simulink model "WorkingModel"  (R2023b)
settings: Solver=FixedStepDiscrete  StartTime=0.0  StopTime=param_sim_time  FixedStep=1/fs  MaxStep=1/fs  RelTol=1e-3
undefined symbols (not defined in the file): analyses, fdesignblkfcn, fs, gcbh, param_tot_samples
libraries: dspstat3 x13, SCGAnalysis_SignalGenerationLib x2
(part 10 of 20)

== system WorkingModel/SCG Analysis/Enabled SCG Analysis Subsystem/All Signals Signal Metric Characterization/SCG S2 3DMechAxis Signal Metric Characterization/Average Signal-to-Noise Ratio Calculator/Average S2 Signal-to-Noise Ratio ==
  r_pos : Inport
  scg_signal : Inport  Port=2
  " " : Constant  Value=s2snr_flag
  Average S2 SNR Calculator : MATLAB Function  TreatAsAtomicUnit=on
  Constant : Constant  Value=fs
  Constant1 : Constant  Value=0
  Switch : Switch  Criteria=u2 > Threshold  AllowDiffInputSizes=on  SaturateOnIntegerOverflow=off  InputSameDT=off
  average_s2snr : Outport
  wires:
  r_pos/1 -> Switch/1
  Constant1/1 -> Switch/3
  " "/1 -> Switch/2
  Constant/1 -> Average S2 SNR Calculator/1(fs)
  scg_signal/1 -> Average S2 SNR Calculator/3(scg_signal)
  Switch/1 -> Average S2 SNR Calculator/2(r_pos)
  Average S2 SNR Calculator/1(average_s2_snr) -> average_s2snr/1

== system WorkingModel/SCG Analysis/Enabled SCG Analysis Subsystem/All Signals Signal Metric Characterization/SCG S2 3DMechAxis Signal Metric Characterization/Average Signal-to-Noise Ratio Calculator/Average S2X Signal-to-Noise Ratio ==
  r_pos : Inport
  scg_signal : Inport  Port=2
  " " : Constant  Value=s2xsnr_flag
  Average S2X SNR Calculator : MATLAB Function  TreatAsAtomicUnit=on
  Constant : Constant  Value=fs
  Constant1 : Constant  Value=0
  Switch : Switch  Criteria=u2 > Threshold  AllowDiffInputSizes=on  SaturateOnIntegerOverflow=off  InputSameDT=off
  average_s2Xsnr : Outport
  wires:
  r_pos/1 -> Switch/1
  Constant1/1 -> Switch/3
  " "/1 -> Switch/2
  Constant/1 -> Average S2X SNR Calculator/1(fs)
  scg_signal/1 -> Average S2X SNR Calculator/3(scg_signal)
  Switch/1 -> Average S2X SNR Calculator/2(r_pos)
  Average S2X SNR Calculator/1(average_s2x_snr) -> average_s2Xsnr/1

== system WorkingModel/SCG Analysis/Enabled SCG Analysis Subsystem/All Signals Signal Metric Characterization/SCG Systolic 3DAntiMechAxis Signal Metric Characterization/Average Signal-to-Noise Ratio Calculator/Average S1 Signal-to-Noise Ratio ==
  r_pos : Inport
  scg_signal : Inport  Port=2
  " " : Constant  Value=s1snr_flag
  Average S1 SNR Calculator : MATLAB Function  TreatAsAtomicUnit=on
  Constant : Constant  Value=fs
  Constant1 : Constant  Value=0
  Switch : Switch  Criteria=u2 > Threshold  AllowDiffInputSizes=on  SaturateOnIntegerOverflow=off  InputSameDT=off
  average_s1snr : Outport
  wires:
  scg_signal/1 -> Average S1 SNR Calculator/3(scg_signal)
  Average S1 SNR Calculator/1(average_s1_snr) -> average_s1snr/1
  Constant/1 -> Average S1 SNR Calculator/1(fs)
  " "/1 -> Switch/2
  Switch/1 -> Average S1 SNR Calculator/2(r_pos)
  r_pos/1 -> Switch/1
  Constant1/1 -> Switch/3

== system WorkingModel/SCG Analysis/Enabled SCG Analysis Subsystem/All Signals Signal Metric Characterization/SCG Systolic 3DAntiMechAxis Signal Metric Characterization/Average Signal-to-Noise Ratio Calculator/Average S1X Signal-to-Noise Ratio ==
  r_pos : Inport
  scg_signal : Inport  Port=2
  " " : Constant  Value=s1xsnr_flag
  Average S1 SNR Amplitude Calculator : MATLAB Function  TreatAsAtomicUnit=on
  Constant : Constant  Value=fs
  Constant1 : Constant  Value=0
  Switch : Switch  Criteria=u2 > Threshold  AllowDiffInputSizes=on  SaturateOnIntegerOverflow=off  InputSameDT=off
  average_s1Xsnr : Outport
  wires:
  Average S1 SNR Amplitude Calculator/1(average_s1x_snr) -> average_s1Xsnr/1
  Switch/1 -> Average S1 SNR Amplitude Calculator/2(r_pos)
  scg_signal/1 -> Average S1 SNR Amplitude Calculator/3(scg_signal)
  Constant/1 -> Average S1 SNR Amplitude Calculator/1(fs)
  " "/1 -> Switch/2
  Constant1/1 -> Switch/3
  r_pos/1 -> Switch/1

== system WorkingModel/SCG Analysis/Enabled SCG Analysis Subsystem/All Signals Signal Metric Characterization/SCG Systolic 3DAntiMechAxis Signal Metric Characterization/Average Signal-to-Noise Ratio Calculator/Average S2 Signal-to-Noise Ratio ==
  r_pos : Inport
  scg_signal : Inport  Port=2
  " " : Constant  Value=s2snr_flag
  Average S2 SNR Calculator : MATLAB Function  TreatAsAtomicUnit=on
  Constant : Constant  Value=fs
  Constant1 : Constant  Value=0
  Switch : Switch  Criteria=u2 > Threshold  AllowDiffInputSizes=on  SaturateOnIntegerOverflow=off  InputSameDT=off
  average_s2snr : Outport
  wires:
  Average S2 SNR Calculator/1(average_s2_snr) -> average_s2snr/1
  Switch/1 -> Average S2 SNR Calculator/2(r_pos)
  scg_signal/1 -> Average S2 SNR Calculator/3(scg_signal)
  Constant/1 -> Average S2 SNR Calculator/1(fs)
  " "/1 -> Switch/2
  Constant1/1 -> Switch/3
  r_pos/1 -> Switch/1

== system WorkingModel/SCG Analysis/Enabled SCG Analysis Subsystem/All Signals Signal Metric Characterization/SCG Systolic 3DAntiMechAxis Signal Metric Characterization/Average Signal-to-Noise Ratio Calculator/Average S2X Signal-to-Noise Ratio ==
  r_pos : Inport
  scg_signal : Inport  Port=2
  " " : Constant  Value=s2xsnr_flag
  Average S2X SNR Calculator : MATLAB Function  TreatAsAtomicUnit=on
  Constant : Constant  Value=fs
  Constant1 : Constant  Value=0
  Switch : Switch  Criteria=u2 > Threshold  AllowDiffInputSizes=on  SaturateOnIntegerOverflow=off  InputSameDT=off
  average_s2Xsnr : Outport
  wires:
  Average S2X SNR Calculator/1(average_s2x_snr) -> average_s2Xsnr/1
  Switch/1 -> Average S2X SNR Calculator/2(r_pos)
  scg_signal/1 -> Average S2X SNR Calculator/3(scg_signal)
  Constant/1 -> Average S2X SNR Calculator/1(fs)
  " "/1 -> Switch/2
  Constant1/1 -> Switch/3
  r_pos/1 -> Switch/1

== system WorkingModel/SCG Analysis/Enabled SCG Analysis Subsystem/All Signals Signal Metric Characterization/SCG Systolic 3DMaxS1p2pProjection Signal Metric Characterization/Average Signal-to-Noise Ratio Calculator/Average S1 Signal-to-Noise Ratio ==
  r_pos : Inport
  scg_signal : Inport  Port=2
  " " : Constant  Value=s1snr_flag
  Average S1 SNR Calculator : MATLAB Function  TreatAsAtomicUnit=on
  Constant : Constant  Value=fs
  Constant1 : Constant  Value=0
  Switch : Switch  Criteria=u2 > Threshold  AllowDiffInputSizes=on  SaturateOnIntegerOverflow=off  InputSameDT=off
  average_s1snr : Outport
  wires:
  Constant1/1 -> Switch/3
  r_pos/1 -> Switch/1
  Switch/1 -> Average S1 SNR Calculator/2(r_pos)
  " "/1 -> Switch/2
  Constant/1 -> Average S1 SNR Calculator/1(fs)
  Average S1 SNR Calculator/1(average_s1_snr) -> average_s1snr/1
  scg_signal/1 -> Average S1 SNR Calculator/3(scg_signal)

== system WorkingModel/SCG Analysis/Enabled SCG Analysis Subsystem/All Signals Signal Metric Characterization/SCG Systolic 3DMaxS1p2pProjection Signal Metric Characterization/Average Signal-to-Noise Ratio Calculator/Average S1X Signal-to-Noise Ratio ==
  r_pos : Inport
  scg_signal : Inport  Port=2
  " " : Constant  Value=s1xsnr_flag
  Average S1 SNR Amplitude Calculator : MATLAB Function  TreatAsAtomicUnit=on
  Constant : Constant  Value=fs
  Constant1 : Constant  Value=0
  Switch : Switch  Criteria=u2 > Threshold  AllowDiffInputSizes=on  SaturateOnIntegerOverflow=off  InputSameDT=off
  average_s1Xsnr : Outport
  wires:
  r_pos/1 -> Switch/1
  Constant1/1 -> Switch/3
  " "/1 -> Switch/2
  Constant/1 -> Average S1 SNR Amplitude Calculator/1(fs)
  scg_signal/1 -> Average S1 SNR Amplitude Calculator/3(scg_signal)
  Switch/1 -> Average S1 SNR Amplitude Calculator/2(r_pos)
  Average S1 SNR Amplitude Calculator/1(average_s1x_snr) -> average_s1Xsnr/1

== system WorkingModel/SCG Analysis/Enabled SCG Analysis Subsystem/All Signals Signal Metric Characterization/SCG Systolic 3DMaxS1p2pProjection Signal Metric Characterization/Average Signal-to-Noise Ratio Calculator/Average S2 Signal-to-Noise Ratio ==
  r_pos : Inport
  scg_signal : Inport  Port=2
  " " : Constant  Value=s2snr_flag
  Average S2 SNR Calculator : MATLAB Function  TreatAsAtomicUnit=on
  Constant : Constant  Value=fs
  Constant1 : Constant  Value=0
  Switch : Switch  Criteria=u2 > Threshold  AllowDiffInputSizes=on  SaturateOnIntegerOverflow=off  InputSameDT=off
  average_s2snr : Outport
  wires:
  r_pos/1 -> Switch/1
  Constant1/1 -> Switch/3
  " "/1 -> Switch/2
  Constant/1 -> Average S2 SNR Calculator/1(fs)
  scg_signal/1 -> Average S2 SNR Calculator/3(scg_signal)
  Switch/1 -> Average S2 SNR Calculator/2(r_pos)
  Average S2 SNR Calculator/1(average_s2_snr) -> average_s2snr/1

== system WorkingModel/SCG Analysis/Enabled SCG Analysis Subsystem/All Signals Signal Metric Characterization/SCG Systolic 3DMaxS1p2pProjection Signal Metric Characterization/Average Signal-to-Noise Ratio Calculator/Average S2X Signal-to-Noise Ratio ==
  r_pos : Inport
  scg_signal : Inport  Port=2
  " " : Constant  Value=s2xsnr_flag
  Average S2X SNR Calculator : MATLAB Function  TreatAsAtomicUnit=on
  Constant : Constant  Value=fs
  Constant1 : Constant  Value=0
  Switch : Switch  Criteria=u2 > Threshold  AllowDiffInputSizes=on  SaturateOnIntegerOverflow=off  InputSameDT=off
  average_s2Xsnr : Outport
  wires:
  r_pos/1 -> Switch/1
  Constant1/1 -> Switch/3
  " "/1 -> Switch/2
  Constant/1 -> Average S2X SNR Calculator/1(fs)
  scg_signal/1 -> Average S2X SNR Calculator/3(scg_signal)
  Switch/1 -> Average S2X SNR Calculator/2(r_pos)
  Average S2X SNR Calculator/1(average_s2x_snr) -> average_s2Xsnr/1

== system WorkingModel/SCG Analysis/Enabled SCG Analysis Subsystem/All Signals Signal Metric Characterization/SCG Systolic 3DMechAxis Signal Metric Characterization/Average Signal-to-Noise Ratio Calculator/Average S1 Signal-to-Noise Ratio ==
  r_pos : Inport
  scg_signal : Inport  Port=2
  " " : Constant  Value=s1snr_flag
  Average S1 SNR Calculator : MATLAB Function  TreatAsAtomicUnit=on
  Constant : Constant  Value=fs
  Constant1 : Constant  Value=0
  Switch : Switch  Criteria=u2 > Threshold  AllowDiffInputSizes=on  SaturateOnIntegerOverflow=off  InputSameDT=off
  average_s1snr : Outport
  wires:
  Constant1/1 -> Switch/3
  r_pos/1 -> Switch/1
  Switch/1 -> Average S1 SNR Calculator/2(r_pos)
  " "/1 -> Switch/2
  Constant/1 -> Average S1 SNR Calculator/1(fs)
  Average S1 SNR Calculator/1(average_s1_snr) -> average_s1snr/1
  scg_signal/1 -> Average S1 SNR Calculator/3(scg_signal)

== system WorkingModel/SCG Analysis/Enabled SCG Analysis Subsystem/All Signals Signal Metric Characterization/SCG Systolic 3DMechAxis Signal Metric Characterization/Average Signal-to-Noise Ratio Calculator/Average S1X Signal-to-Noise Ratio ==
  r_pos : Inport
  scg_signal : Inport  Port=2
  " " : Constant  Value=s1xsnr_flag
  Average S1 SNR Amplitude Calculator : MATLAB Function  TreatAsAtomicUnit=on
  Constant : Constant  Value=fs
  Constant1 : Constant  Value=0
  Switch : Switch  Criteria=u2 > Threshold  AllowDiffInputSizes=on  SaturateOnIntegerOverflow=off  InputSameDT=off
  average_s1Xsnr : Outport
  wires:
  r_pos/1 -> Switch/1
  Constant1/1 -> Switch/3
  " "/1 -> Switch/2
  Constant/1 -> Average S1 SNR Amplitude Calculator/1(fs)
  scg_signal/1 -> Average S1 SNR Amplitude Calculator/3(scg_signal)
  Switch/1 -> Average S1 SNR Amplitude Calculator/2(r_pos)
  Average S1 SNR Amplitude Calculator/1(average_s1x_snr) -> average_s1Xsnr/1

== system WorkingModel/SCG Analysis/Enabled SCG Analysis Subsystem/All Signals Signal Metric Characterization/SCG Systolic 3DMechAxis Signal Metric Characterization/Average Signal-to-Noise Ratio Calculator/Average S2 Signal-to-Noise Ratio ==
  r_pos : Inport
  scg_signal : Inport  Port=2
  " " : Constant  Value=s2snr_flag
  Average S2 SNR Calculator : MATLAB Function  TreatAsAtomicUnit=on
  Constant : Constant  Value=fs
  Constant1 : Constant  Value=0
  Switch : Switch  Criteria=u2 > Threshold  AllowDiffInputSizes=on  SaturateOnIntegerOverflow=off  InputSameDT=off
  average_s2snr : Outport
  wires:
  r_pos/1 -> Switch/1
  Constant1/1 -> Switch/3
  " "/1 -> Switch/2
  Constant/1 -> Average S2 SNR Calculator/1(fs)
  scg_signal/1 -> Average S2 SNR Calculator/3(scg_signal)
  Switch/1 -> Average S2 SNR Calculator/2(r_pos)
  Average S2 SNR Calculator/1(average_s2_snr) -> average_s2snr/1

== system WorkingModel/SCG Analysis/Enabled SCG Analysis Subsystem/All Signals Signal Metric Characterization/SCG Systolic 3DMechAxis Signal Metric Characterization/Average Signal-to-Noise Ratio Calculator/Average S2X Signal-to-Noise Ratio ==
  r_pos : Inport
  scg_signal : Inport  Port=2
  " " : Constant  Value=s2xsnr_flag
  Average S2X SNR Calculator : MATLAB Function  TreatAsAtomicUnit=on
  Constant : Constant  Value=fs
  Constant1 : Constant  Value=0
  Switch : Switch  Criteria=u2 > Threshold  AllowDiffInputSizes=on  SaturateOnIntegerOverflow=off  InputSameDT=off
  average_s2Xsnr : Outport
  wires:
  r_pos/1 -> Switch/1
  Constant1/1 -> Switch/3
  " "/1 -> Switch/2
  Constant/1 -> Average S2X SNR Calculator/1(fs)
  scg_signal/1 -> Average S2X SNR Calculator/3(scg_signal)
  Switch/1 -> Average S2X SNR Calculator/2(r_pos)
  Average S2X SNR Calculator/1(average_s2x_snr) -> average_s2Xsnr/1

== system WorkingModel/SCG Analysis/Enabled SCG Analysis Subsystem/All Signals Signal Metric Characterization/SCG Systolic 3DMinS1p2pProjection Signal Metric Characterization/Average Signal-to-Noise Ratio Calculator/Average S1 Signal-to-Noise Ratio ==
  r_pos : Inport
  scg_signal : Inport  Port=2
  " " : Constant  Value=s1snr_flag
  Average S1 SNR Calculator : MATLAB Function  TreatAsAtomicUnit=on
  Constant : Constant  Value=fs
  Constant1 : Constant  Value=0
  Switch : Switch  Criteria=u2 > Threshold  AllowDiffInputSizes=on  SaturateOnIntegerOverflow=off  InputSameDT=off
  average_s1snr : Outport
  wires:
  scg_signal/1 -> Average S1 SNR Calculator/3(scg_signal)
  Average S1 SNR Calculator/1(average_s1_snr) -> average_s1snr/1
  Constant/1 -> Average S1 SNR Calculator/1(fs)
  " "/1 -> Switch/2
  Switch/1 -> Average S1 SNR Calculator/2(r_pos)
  r_pos/1 -> Switch/1
  Constant1/1 -> Switch/3

== system WorkingModel/SCG Analysis/Enabled SCG Analysis Subsystem/All Signals Signal Metric Characterization/SCG Systolic 3DMinS1p2pProjection Signal Metric Characterization/Average Signal-to-Noise Ratio Calculator/Average S1X Signal-to-Noise Ratio ==
  r_pos : Inport
  scg_signal : Inport  Port=2
  " " : Constant  Value=s1xsnr_flag
  Average S1 SNR Amplitude Calculator : MATLAB Function  TreatAsAtomicUnit=on
  Constant : Constant  Value=fs
  Constant1 : Constant  Value=0
  Switch : Switch  Criteria=u2 > Threshold  AllowDiffInputSizes=on  SaturateOnIntegerOverflow=off  InputSameDT=off
  average_s1Xsnr : Outport
  wires:
  Average S1 SNR Amplitude Calculator/1(average_s1x_snr) -> average_s1Xsnr/1
  Switch/1 -> Average S1 SNR Amplitude Calculator/2(r_pos)
  scg_signal/1 -> Average S1 SNR Amplitude Calculator/3(scg_signal)
  Constant/1 -> Average S1 SNR Amplitude Calculator/1(fs)
  " "/1 -> Switch/2
  Constant1/1 -> Switch/3
  r_pos/1 -> Switch/1

== system WorkingModel/SCG Analysis/Enabled SCG Analysis Subsystem/All Signals Signal Metric Characterization/SCG Systolic 3DMinS1p2pProjection Signal Metric Characterization/Average Signal-to-Noise Ratio Calculator/Average S2 Signal-to-Noise Ratio ==
  r_pos : Inport
  scg_signal : Inport  Port=2
  " " : Constant  Value=s2snr_flag
  Average S2 SNR Calculator : MATLAB Function  TreatAsAtomicUnit=on
  Constant : Constant  Value=fs
  Constant1 : Constant  Value=0
  Switch : Switch  Criteria=u2 > Threshold  AllowDiffInputSizes=on  SaturateOnIntegerOverflow=off  InputSameDT=off
  average_s2snr : Outport
  wires:
  Average S2 SNR Calculator/1(average_s2_snr) -> average_s2snr/1
  Switch/1 -> Average S2 SNR Calculator/2(r_pos)
  scg_signal/1 -> Average S2 SNR Calculator/3(scg_signal)
  Constant/1 -> Average S2 SNR Calculator/1(fs)
  " "/1 -> Switch/2
  Constant1/1 -> Switch/3
  r_pos/1 -> Switch/1

== system WorkingModel/SCG Analysis/Enabled SCG Analysis Subsystem/All Signals Signal Metric Characterization/SCG Systolic 3DMinS1p2pProjection Signal Metric Characterization/Average Signal-to-Noise Ratio Calculator/Average S2X Signal-to-Noise Ratio ==
  r_pos : Inport
  scg_signal : Inport  Port=2
  " " : Constant  Value=s2xsnr_flag
  Average S2X SNR Calculator : MATLAB Function  TreatAsAtomicUnit=on
  Constant : Constant  Value=fs
  Constant1 : Constant  Value=0
  Switch : Switch  Criteria=u2 > Threshold  AllowDiffInputSizes=on  SaturateOnIntegerOverflow=off  InputSameDT=off
  average_s2Xsnr : Outport
  wires:
  Average S2X SNR Calculator/1(average_s2x_snr) -> average_s2Xsnr/1
  Switch/1 -> Average S2X SNR Calculator/2(r_pos)
  scg_signal/1 -> Average S2X SNR Calculator/3(scg_signal)
  Constant/1 -> Average S2X SNR Calculator/1(fs)
  " "/1 -> Switch/2
  Constant1/1 -> Switch/3
  r_pos/1 -> Switch/1

== system WorkingModel/SCG Analysis/Enabled SCG Analysis Subsystem/All Signals Signal Metric Characterization/SCG X Signal Metric Characterization/Average Signal-to-Noise Ratio Calculator/Average S1 Signal-to-Noise Ratio ==
  r_pos : Inport
  scg_signal : Inport  Port=2
  " " : Constant  Value=s1snr_flag
  Average S1 SNR Calculator : MATLAB Function  TreatAsAtomicUnit=on
  Constant : Constant  Value=fs
  Constant1 : Constant  Value=0
  Switch : Switch  Criteria=u2 > Threshold  AllowDiffInputSizes=on  SaturateOnIntegerOverflow=off  InputSameDT=off
  average_s1snr : Outport
  wires:
  scg_signal/1 -> Average S1 SNR Calculator/3(scg_signal)
  Average S1 SNR Calculator/1(average_s1_snr) -> average_s1snr/1
  Constant/1 -> Average S1 SNR Calculator/1(fs)
  " "/1 -> Switch/2
  Switch/1 -> Average S1 SNR Calculator/2(r_pos)
  r_pos/1 -> Switch/1
  Constant1/1 -> Switch/3

== system WorkingModel/SCG Analysis/Enabled SCG Analysis Subsystem/All Signals Signal Metric Characterization/SCG X Signal Metric Characterization/Average Signal-to-Noise Ratio Calculator/Average S1X Signal-to-Noise Ratio ==
  r_pos : Inport
  scg_signal : Inport  Port=2
  " " : Constant  Value=s1xsnr_flag
  Average S1 SNR Amplitude Calculator : MATLAB Function  TreatAsAtomicUnit=on
  Constant : Constant  Value=fs
  Constant1 : Constant  Value=0
  Switch : Switch  Criteria=u2 > Threshold  AllowDiffInputSizes=on  SaturateOnIntegerOverflow=off  InputSameDT=off
  average_s1Xsnr : Outport
  wires:
  Average S1 SNR Amplitude Calculator/1(average_s1x_snr) -> average_s1Xsnr/1
  Switch/1 -> Average S1 SNR Amplitude Calculator/2(r_pos)
  scg_signal/1 -> Average S1 SNR Amplitude Calculator/3(scg_signal)
  Constant/1 -> Average S1 SNR Amplitude Calculator/1(fs)
  " "/1 -> Switch/2
  Constant1/1 -> Switch/3
  r_pos/1 -> Switch/1

== system WorkingModel/SCG Analysis/Enabled SCG Analysis Subsystem/All Signals Signal Metric Characterization/SCG X Signal Metric Characterization/Average Signal-to-Noise Ratio Calculator/Average S2 Signal-to-Noise Ratio ==
  r_pos : Inport
  scg_signal : Inport  Port=2
  " " : Constant  Value=s2snr_flag
  Average S2 SNR Calculator : MATLAB Function  TreatAsAtomicUnit=on
  Constant : Constant  Value=fs
  Constant1 : Constant  Value=0
  Switch : Switch  Criteria=u2 > Threshold  AllowDiffInputSizes=on  SaturateOnIntegerOverflow=off  InputSameDT=off
  average_s2snr : Outport
  wires:
  Average S2 SNR Calculator/1(average_s2_snr) -> average_s2snr/1
  Switch/1 -> Average S2 SNR Calculator/2(r_pos)
  scg_signal/1 -> Average S2 SNR Calculator/3(scg_signal)
  Constant/1 -> Average S2 SNR Calculator/1(fs)
  " "/1 -> Switch/2
  Constant1/1 -> Switch/3
  r_pos/1 -> Switch/1

== system WorkingModel/SCG Analysis/Enabled SCG Analysis Subsystem/All Signals Signal Metric Characterization/SCG X Signal Metric Characterization/Average Signal-to-Noise Ratio Calculator/Average S2X Signal-to-Noise Ratio ==
  r_pos : Inport
  scg_signal : Inport  Port=2
  " " : Constant  Value=s2xsnr_flag
  Average S2X SNR Calculator : MATLAB Function  TreatAsAtomicUnit=on
  Constant : Constant  Value=fs
  Constant1 : Constant  Value=0
  Switch : Switch  Criteria=u2 > Threshold  AllowDiffInputSizes=on  SaturateOnIntegerOverflow=off  InputSameDT=off
  average_s2Xsnr : Outport
  wires:
  Average S2X SNR Calculator/1(average_s2x_snr) -> average_s2Xsnr/1
  Switch/1 -> Average S2X SNR Calculator/2(r_pos)
  scg_signal/1 -> Average S2X SNR Calculator/3(scg_signal)
  Constant/1 -> Average S2X SNR Calculator/1(fs)
  " "/1 -> Switch/2
  Constant1/1 -> Switch/3
  r_pos/1 -> Switch/1

== system WorkingModel/SCG Analysis/Enabled SCG Analysis Subsystem/All Signals Signal Metric Characterization/SCG Y Signal Metric Characterization/Average Signal-to-Noise Ratio Calculator/Average S1 Signal-to-Noise Ratio ==
  r_pos : Inport
  scg_signal : Inport  Port=2
  " " : Constant  Value=s1snr_flag
  Average S1 SNR Calculator : MATLAB Function  TreatAsAtomicUnit=on
  Constant : Constant  Value=fs
  Constant1 : Constant  Value=0
  Switch : Switch  Criteria=u2 > Threshold  AllowDiffInputSizes=on  SaturateOnIntegerOverflow=off  InputSameDT=off
  average_s1snr : Outport
  wires:
  Constant1/1 -> Switch/3
  r_pos/1 -> Switch/1
  Switch/1 -> Average S1 SNR Calculator/2(r_pos)
  " "/1 -> Switch/2
  Constant/1 -> Average S1 SNR Calculator/1(fs)
  Average S1 SNR Calculator/1(average_s1_snr) -> average_s1snr/1
  scg_signal/1 -> Average S1 SNR Calculator/3(scg_signal)

== system WorkingModel/SCG Analysis/Enabled SCG Analysis Subsystem/All Signals Signal Metric Characterization/SCG Y Signal Metric Characterization/Average Signal-to-Noise Ratio Calculator/Average S1X Signal-to-Noise Ratio ==
  r_pos : Inport
  scg_signal : Inport  Port=2
  " " : Constant  Value=s1xsnr_flag
  Average S1 SNR Amplitude Calculator : MATLAB Function  TreatAsAtomicUnit=on
  Constant : Constant  Value=fs
  Constant1 : Constant  Value=0
  Switch : Switch  Criteria=u2 > Threshold  AllowDiffInputSizes=on  SaturateOnIntegerOverflow=off  InputSameDT=off
  average_s1Xsnr : Outport
  wires:
  r_pos/1 -> Switch/1
  Constant1/1 -> Switch/3
  " "/1 -> Switch/2
  Constant/1 -> Average S1 SNR Amplitude Calculator/1(fs)
  scg_signal/1 -> Average S1 SNR Amplitude Calculator/3(scg_signal)
  Switch/1 -> Average S1 SNR Amplitude Calculator/2(r_pos)
  Average S1 SNR Amplitude Calculator/1(average_s1x_snr) -> average_s1Xsnr/1

== system WorkingModel/SCG Analysis/Enabled SCG Analysis Subsystem/All Signals Signal Metric Characterization/SCG Y Signal Metric Characterization/Average Signal-to-Noise Ratio Calculator/Average S2 Signal-to-Noise Ratio ==
  r_pos : Inport
  scg_signal : Inport  Port=2
  " " : Constant  Value=s2snr_flag
  Average S2 SNR Calculator : MATLAB Function  TreatAsAtomicUnit=on
  Constant : Constant  Value=fs
  Constant1 : Constant  Value=0
  Switch : Switch  Criteria=u2 > Threshold  AllowDiffInputSizes=on  SaturateOnIntegerOverflow=off  InputSameDT=off
  average_s2snr : Outport
  wires:
  r_pos/1 -> Switch/1
  Constant1/1 -> Switch/3
  " "/1 -> Switch/2
  Constant/1 -> Average S2 SNR Calculator/1(fs)
  scg_signal/1 -> Average S2 SNR Calculator/3(scg_signal)
  Switch/1 -> Average S2 SNR Calculator/2(r_pos)
  Average S2 SNR Calculator/1(average_s2_snr) -> average_s2snr/1

== system WorkingModel/SCG Analysis/Enabled SCG Analysis Subsystem/All Signals Signal Metric Characterization/SCG Y Signal Metric Characterization/Average Signal-to-Noise Ratio Calculator/Average S2X Signal-to-Noise Ratio ==
  r_pos : Inport
  scg_signal : Inport  Port=2
  " " : Constant  Value=s2xsnr_flag
  Average S2X SNR Calculator : MATLAB Function  TreatAsAtomicUnit=on
  Constant : Constant  Value=fs
  Constant1 : Constant  Value=0
  Switch : Switch  Criteria=u2 > Threshold  AllowDiffInputSizes=on  SaturateOnIntegerOverflow=off  InputSameDT=off
  average_s2Xsnr : Outport
  wires:
  r_pos/1 -> Switch/1
  Constant1/1 -> Switch/3
  " "/1 -> Switch/2
  Constant/1 -> Average S2X SNR Calculator/1(fs)
  scg_signal/1 -> Average S2X SNR Calculator/3(scg_signal)
  Switch/1 -> Average S2X SNR Calculator/2(r_pos)
  Average S2X SNR Calculator/1(average_s2x_snr) -> average_s2Xsnr/1

== system WorkingModel/SCG Analysis/Enabled SCG Analysis Subsystem/All Signals Signal Metric Characterization/SCG Z Signal Metric Characterization/Average Signal-to-Noise Ratio Calculator/Average S1 Signal-to-Noise Ratio ==
  r_pos : Inport
  scg_signal : Inport  Port=2
  " " : Constant  Value=s1snr_flag
  Average S1 SNR Calculator : MATLAB Function  TreatAsAtomicUnit=on
  Constant : Constant  Value=fs
  Constant1 : Constant  Value=0
  Switch : Switch  Criteria=u2 > Threshold  AllowDiffInputSizes=on  SaturateOnIntegerOverflow=off  InputSameDT=off
  average_s1snr : Outport
  wires:
  scg_signal/1 -> Average S1 SNR Calculator/3(scg_signal)
  Average S1 SNR Calculator/1(average_s1_snr) -> average_s1snr/1
  Constant/1 -> Average S1 SNR Calculator/1(fs)
  " "/1 -> Switch/2
  Switch/1 -> Average S1 SNR Calculator/2(r_pos)
  r_pos/1 -> Switch/1
  Constant1/1 -> Switch/3

== system WorkingModel/SCG Analysis/Enabled SCG Analysis Subsystem/All Signals Signal Metric Characterization/SCG Z Signal Metric Characterization/Average Signal-to-Noise Ratio Calculator/Average S1X Signal-to-Noise Ratio ==
  r_pos : Inport
  scg_signal : Inport  Port=2
  " " : Constant  Value=s1xsnr_flag
  Average S1 SNR Amplitude Calculator : MATLAB Function  TreatAsAtomicUnit=on
  Constant : Constant  Value=fs
  Constant1 : Constant  Value=0
  Switch : Switch  Criteria=u2 > Threshold  AllowDiffInputSizes=on  SaturateOnIntegerOverflow=off  InputSameDT=off
  average_s1Xsnr : Outport
  wires:
  Average S1 SNR Amplitude Calculator/1(average_s1x_snr) -> average_s1Xsnr/1
  Switch/1 -> Average S1 SNR Amplitude Calculator/2(r_pos)
  scg_signal/1 -> Average S1 SNR Amplitude Calculator/3(scg_signal)
  Constant/1 -> Average S1 SNR Amplitude Calculator/1(fs)
  " "/1 -> Switch/2
  Constant1/1 -> Switch/3
  r_pos/1 -> Switch/1

== system WorkingModel/SCG Analysis/Enabled SCG Analysis Subsystem/All Signals Signal Metric Characterization/SCG Z Signal Metric Characterization/Average Signal-to-Noise Ratio Calculator/Average S2 Signal-to-Noise Ratio ==
  r_pos : Inport
  scg_signal : Inport  Port=2
  " " : Constant  Value=s2snr_flag
  Average S2 SNR Calculator : MATLAB Function  TreatAsAtomicUnit=on
  Constant : Constant  Value=fs
  Constant1 : Constant  Value=0
  Switch : Switch  Criteria=u2 > Threshold  AllowDiffInputSizes=on  SaturateOnIntegerOverflow=off  InputSameDT=off
  average_s2snr : Outport
  wires:
  Average S2 SNR Calculator/1(average_s2_snr) -> average_s2snr/1
  Switch/1 -> Average S2 SNR Calculator/2(r_pos)
  scg_signal/1 -> Average S2 SNR Calculator/3(scg_signal)
  Constant/1 -> Average S2 SNR Calculator/1(fs)
  " "/1 -> Switch/2
  Constant1/1 -> Switch/3
  r_pos/1 -> Switch/1

== system WorkingModel/SCG Analysis/Enabled SCG Analysis Subsystem/All Signals Signal Metric Characterization/SCG Z Signal Metric Characterization/Average Signal-to-Noise Ratio Calculator/Average S2X Signal-to-Noise Ratio ==
  r_pos : Inport
  scg_signal : Inport  Port=2
  " " : Constant  Value=s2xsnr_flag
  Average S2X SNR Calculator : MATLAB Function  TreatAsAtomicUnit=on
  Constant : Constant  Value=fs
  Constant1 : Constant  Value=0
  Switch : Switch  Criteria=u2 > Threshold  AllowDiffInputSizes=on  SaturateOnIntegerOverflow=off  InputSameDT=off
  average_s2Xsnr : Outport
  wires:
  Average S2X SNR Calculator/1(average_s2x_snr) -> average_s2Xsnr/1
  Switch/1 -> Average S2X SNR Calculator/2(r_pos)
  scg_signal/1 -> Average S2X SNR Calculator/3(scg_signal)
  Constant/1 -> Average S2X SNR Calculator/1(fs)
  " "/1 -> Switch/2
  Constant1/1 -> Switch/3
  r_pos/1 -> Switch/1

== matlab function WorkingModel/SCG Analysis/Enabled SCG Analysis Subsystem/Signal Generation/3D Projections/MATLAB Function6 ==
  data: scg_xyz input; el_scg input size=[1]; projection output size=[param_tot_samples 1]; az_scg input size=[1]
function projection = slk_axis_projection(scg_xyz, el_scg, az_scg)

el_mat = el_scg;
az_mat = -1*az_scg;

[xhat_mat, yhat_mat, zhat_mat] = sph2cart(az_mat*pi/180,el_mat*pi/180,1);
% Converting to the SCG convention reference frame (this depends on the accelerometer and its placement orientation! - they should be such that they match the conventional SCG reference frame).
xhat_scg = xhat_mat;
yhat_scg = zhat_mat;
zhat_scg = -1*yhat_mat;

projection_axis = [xhat_scg yhat_scg zhat_scg];
    
projection = zeros(size(scg_xyz,1),1);
    
for i=1:size(scg_xyz,1)
    
    projection(i) = dot(scg_xyz(i,:),projection_axis);
    
end

figure;
ax = [0 0 0 0];

ax(1) = subplot(4,1,1); plot(scg_xyz(:,1),'b'); title('x'); box off; ylabel('Acceleration (mg)');
ax(2) = subplot(4,1,2); plot(scg_xyz(:,2),'b'); title('y'); box off; ylabel('Acceleration (mg)');
ax(3) = subplot(4,1,3); plot(scg_xyz(:,3),'b'); title('z'); box off; ylabel('Acceleration (mg)');
ax(4) = subplot(4,1,4); plot(projection,'g'); title('Systolic Max S2 P2P Axis Projection'); box off; ylabel('Acceleration (mg)');
xlabel('Sample no.')
linkaxes(ax,'xy')
end

== matlab function WorkingModel/SCG Analysis/Enabled SCG Analysis Subsystem/Signal Generation/3D Projections/MATLAB Function7 ==
  data: scg_xyz input; el_scg input size=[1]; projection output size=[param_tot_samples 1]; az_scg input size=[1]
function projection = slk_axis_projection(scg_xyz, el_scg, az_scg)

el_mat = el_scg;
az_mat = -1*az_scg;

[xhat_mat, yhat_mat, zhat_mat] = sph2cart(az_mat*pi/180,el_mat*pi/180,1);
% Converting to the SCG convention reference frame (this depends on the accelerometer and its placement orientation! - they should be such that they match the conventional SCG reference frame).
xhat_scg = xhat_mat;
yhat_scg = zhat_mat;
zhat_scg = -1*yhat_mat;

projection_axis = [xhat_scg yhat_scg zhat_scg];
    
projection = zeros(size(scg_xyz,1),1);
    
for i=1:size(scg_xyz,1)
    
    projection(i) = dot(scg_xyz(i,:),projection_axis);
    
end

figure;
ax = [0 0 0 0];

ax(1) = subplot(4,1,1); plot(scg_xyz(:,1),'b'); title('x'); box off; ylabel('Acceleration (mg)');
ax(2) = subplot(4,1,2); plot(scg_xyz(:,2),'b'); title('y'); box off; ylabel('Acceleration (mg)');
ax(3) = subplot(4,1,3); plot(scg_xyz(:,3),'b'); title('z'); box off; ylabel('Acceleration (mg)');
ax(4) = subplot(4,1,4); plot(projection,'r'); title('Systolic Min S2 P2P Axis Projection'); box off; ylabel('Acceleration (mg)');
xlabel('Sample no.')
linkaxes(ax,'xy')
end

== matlab function WorkingModel/SCG Analysis/Enabled SCG Analysis Subsystem/All Signals Signal Metric Characterization/SCG S2 3DAntiMechAxis Signal Metric Characterization/Average S2 peak-to-peak Amplitude Calculator/Average S2p2p Amplitude Calculator ==
  data: fs input; r_pos input; scg_signal input; average_s2p2pamp output size=[1]
function average_s2p2pamp = slk_average_s2p2pamp_calculator(fs, r_pos, scg_signal)
% Function to calculate the average (mean) S2 peak-to-peak amplitude from an SCG input signal.

coder.extrinsic('sgtitle'); % Needed later for plotting.

num_cycles = length(r_pos);

s2p2pamp = zeros(1,num_cycles - 1); % Pre-initialization for speed.
s2_peak_pos = zeros(1,num_cycles - 1); 
s2_trough_pos = zeros(1,num_cycles - 1); 
s2_search_window_lims = [0.25*fs 0.5*fs]; % The window initially used to search for the S2 peak within that cycle.

for i = 1:num_cycles - 1 % The last heart cycle isn't considered because there's a signficant change that its S2 complex has been cut-off.
    
    cycle = scg_signal(r_pos(i):r_pos(i+1)); % The current heart cycle.
    
    s2_search_window = cycle(s2_search_window_lims(1):s2_search_window_lims(2)); % Defining the window where to search for the S2 peak.
    s2_peak_pos(i) = r_pos(i) + s2_search_window_lims(1) + find(s2_search_window==max(s2_search_window)); % Identifying the S2 peak.
    s2_trough_pos(i) = r_pos(i) + s2_search_window_lims(1) + find(s2_search_window==min(s2_search_window)); % Identifying the S2 trough.
    s2p2pamp(i)= scg_signal(s2_peak_pos(i)) - scg_signal(s2_trough_pos(i));
    
end

average_s2p2pamp = mean(s2p2pamp);

%% Plotting.

figure;
sgtitle('SCG S2 AntiMechAxis')
ax = [0 0]; % Pre-initialization

% Labelled SCG.
t = 0:1/fs:(length(scg_signal)-1)/fs;

ax(1) = subplot(2,1,1);
plot(t,scg_signal); hold on
plot((s2_peak_pos-1)/fs, scg_signal(s2_peak_pos), 'ro') % Plotting the peaks.
plot((s2_trough_pos-1)/fs, scg_signal(s2_trough_pos), 'bo') % Plotting the troughs.
ylim([min(scg_signal)-10 max(scg_signal)+10]);

% Green Vertical Lines to Denote R peak Positions.
for i = 1:num_cycles
    plot([(r_pos(i) - 1)/fs (r_pos(i) - 1)/fs],[min(scg_signal)-10 max(scg_signal)+10],'g--')
end

title('Labelled S2 Peaks + Troughs')
xlabel('Time (sec)')
ylabel('Acceleration (mg)')
box off

%% S2 p2p Amplitude Evolution.
ax(2) = subplot(2,1,2);
plot((((s2_peak_pos + s2_trough_pos)/2) - 1)/fs, s2p2pamp,'.-'); hold on % Plotting the S2 P2P Amp. at the timepoints given by the midpoint between the detected S2 peaks and troughs.
xlabel('Time (sec)')
ylabel('Peak-to-Peak Amplitude (mg)')
title('S2 P2P Amplitude Evolution');
plot([0 (r_pos(end)-1)/fs], [average_s2p2pamp average_s2p2pamp],'r--') % Plotting the average S2 P2P Amp.
box off

linkaxes(ax,'x')

end

== matlab function WorkingModel/SCG Analysis/Enabled SCG Analysis Subsystem/All Signals Signal Metric Characterization/SCG S2 3DAntiMechAxis Signal Metric Characterization/Average Signal-to-Noise Ratio Calculator/Average S1 Signal-to-Noise Ratio/Average S1 SNR Calculator ==
  data: fs input size=[1]; r_pos input; scg_signal input; average_s1_snr output size=[1]
function average_s1_snr = slk_average_s1snr_calculator(fs, r_pos, scg_signal)
% Function to calculate the average (mean) S1 signal-to-noise ratio from an SCG input signal, where:
% Signal = S1 complex
% Noise = rest of cycle

% The signal-to-noise ratio is considered to be the ratio of
% root-mean-square values of the signal and the noise.

if r_pos
    
    num_cycles = length(r_pos);
    
    s1snr = zeros(1,num_cycles); % Pre-initialization for speed.
    
    for i = 1:num_cycles - 1
        signal = scg_signal(r_pos(i):r_pos(i) + 0.2*fs); % The signal is the S1 complex.
        noise = scg_signal(r_pos(i) + 0.2*fs + 1:r_pos(i+1)); % The rest of the cycle is the noise.
        s1snr(i) = rms(signal)/rms(noise); % SnR is the ratio of rms(signal) to rms (noise).
    end
    
    average_s1_snr = mean(s1snr);
    
else
    
    average_s1_snr = nan;
   
end

== matlab function WorkingModel/SCG Analysis/Enabled SCG Analysis Subsystem/All Signals Signal Metric Characterization/SCG S2 3DAntiMechAxis Signal Metric Characterization/Average Signal-to-Noise Ratio Calculator/Average S1X Signal-to-Noise Ratio/Average S1 SNR Amplitude Calculator ==
  data: fs input size=[1]; r_pos input; scg_signal input; average_s1x_snr output size=[1]
function average_s1x_snr = slk_average_s1xsnr_calculator(fs, r_pos, scg_signal)
% Function to calculate the average (mean) S1 signal-to-noise ratio from an SCG input signal, where:
% Signal = S1 complex
% Noise = rest of cycle EXCEPT the S2 complex

% The signal-to-noise ratio is considered to be the ratio of
% root-mean-square values of the signal and the noise.
    
num_cycles = length(r_pos);
s2_search_window_lims = [0.05*fs 0.3*fs]; % The window initially used to search for the S2 peak within the 'noise' segment.
s2_excise_window = fs*0.1; % The window length centered about the S2 peak (in samples) used to excise the S2 complex.

s1xsnr = zeros(1,num_cycles); % Pre-initialization for speed.

for i = 1:num_cycles - 1
    signal = scg_signal(r_pos(i):r_pos(i) + 0.2*fs); % The signal is the S1 complex.
 
    % Removing the S2 complex from the rest of the cycle.
    noise = scg_signal(1 + r_pos(i) + 0.2*fs:r_pos(i+1)); % Rest of the cycle.
    s2_search_window = noise(s2_search_window_lims(1):s2_search_window_lims(2)); % Defining the window where to search for the S2 peak.
    s2peak = s2_search_window_lims(1) + find(abs(s2_search_window) == max(abs(s2_search_window))); % Identifying the S2 peak within "noise".
    noise(s2peak(1) - s2_excise_window/2 : s2peak(1) + s2_excise_window/2) = []; % Removing the S2 complex.
    
    s1xsnr(i) = rms(signal)/rms(noise); % SnR is the ratio of rms(signal) to rms (noise).   
end

average_s1x_snr = mean(s1xsnr);

end

== matlab function WorkingModel/SCG Analysis/Enabled SCG Analysis Subsystem/All Signals Signal Metric Characterization/SCG S2 3DAntiMechAxis Signal Metric Characterization/Average Signal-to-Noise Ratio Calculator/Average S2 Signal-to-Noise Ratio/Average S2 SNR Calculator ==
  data: fs input size=[1]; r_pos input; scg_signal input; average_s2_snr output size=[1]
function average_s2_snr = slk_average_s2snr_calculator(fs, r_pos, scg_signal)
% Function to calculate the average (mean) S2 signal-to-noise ratio from an SCG input signal, where:
% Signal = S2 complex
% Noise = rest of cycle (including the S1 complex)

% The signal-to-noise ratio is considered to be the ratio of root-mean-square values of the signal and the noise.
    
num_cycles = length(r_pos);
s2_search_window_lims = [0.25*fs 0.5*fs]; % The window initially used to search for the S2 peak within that cycle.
s2_identify_window = fs*0.15; % The window length centered about the S2 peak (in samples) used to identify the S2 complex.

s2_snr = zeros(1,num_cycles); % Pre-initialization for speed.

for i = 1:num_cycles - 1 % The last cycle isn't considered because there's a good chance it's cut off.
   
    cycle = scg_signal(r_pos(i):r_pos(i+1)); % The current heart cycle.

    s2_search_window = cycle(s2_search_window_lims(1):s2_search_window_lims(2)); % Defining the window where to search for the S2 peak.
    s2peak = s2_search_window_lims(1) + find(abs(s2_search_window)==max(abs(s2_search_window))); % Identifying the S2 peak within 'cycle'.
    
    signal = cycle(s2peak(1) - s2_identify_window/2 : s2peak(1) + s2_identify_window/2); % The S2 complex is the signal.
    noise = cycle;
    noise(s2peak(1) - s2_identify_window/2 : s2peak(1) + s2_identify_window/2)= []; % Defining the noise as everything except the S2 complex.

    s2_snr(i) = rms(signal)/rms(noise);
    
end

average_s2_snr = mean(s2_snr);

end

== matlab function WorkingModel/SCG Analysis/Enabled SCG Analysis Subsystem/All Signals Signal Metric Characterization/SCG S2 3DAntiMechAxis Signal Metric Characterization/Average Signal-to-Noise Ratio Calculator/Average S2X Signal-to-Noise Ratio/Average S2X SNR Calculator ==
  data: fs input size=[1]; r_pos input; scg_signal input; average_s2x_snr output size=[1]
function average_s2x_snr = slk_average_s2xsnr_calculator(fs, r_pos, scg_signal)
% Function to calculate the average (mean) S2 signal-to-noise ratio from an SCG input signal, where:
% Signal = S2 complex
% Noise = rest of cycle EXCLUDING the S1 complex

% The signal-to-noise ratio is considered to be the ratio of root-mean-square values of the signal and the noise.
    
num_cycles = length(r_pos);
s1_excise_window_lims = [1 0.2*fs]; % The window used to excise the S1 complex from the noise.
s2_search_window_lims = [0.25*fs 0.5*fs]; % The window initially used to search for the S2 peak within that cycle.
s2_identify_window = fs*0.15; % The window length centered about the S2 peak (in samples) used to identify the S2 complex.

s2_snr = zeros(1,num_cycles); % Pre-initialization for speed.

for i = 1:num_cycles - 1
   
    cycle = scg_signal(r_pos(i):r_pos(i+1)); % The current heart cycle.

    s2_search_window = cycle(s2_search_window_lims(1):s2_search_window_lims(2)); % Defining the window where to search for the S2 peak.
    s2peak = s2_search_window_lims(1) + find(abs(s2_search_window) == max(abs(s2_search_window))); % Identifying the S2 peak within 'cycle'.
    
    signal = cycle(s2peak(1) - s2_identify_window/2 : s2peak(1) + s2_identify_window/2); % The S2 complex is the signal.
    noise = cycle;
    noise(s2peak(1) - s2_identify_window/2 : s2peak(1) + s2_identify_window/2)= []; % Removing the S2 complex from the noise.
    noise(s1_excise_window_lims(1):s1_excise_window_lims(2))= [];

    s2_snr(i) = rms(signal)/rms(noise);
    
end

average_s2x_snr = mean(s2_snr);

end
